simulink model "ejercicio"  (Simulink 5.0)
settings: Solver=ode45  StartTime=0.0  StopTime=75.6  RelTol=1e-3
undefined symbols (not defined in the file): Gama
settings Model: LastModifiedBy=Administrador  RTWOptions="-aEnforceIntegerDowncast=1 -aExtMode=0 -aExtModeTesting=0 -aFoldNonRolledExpr=1 -aForceParamTrailComments=0 -aGenerateComments=1 -aGenerateReport=0 -aIgnoreCustomStorageClasses=1 -aIncDataTypeInIds=0 -aIncHierarchyInIds=0 -aInlineInvariantSignals=0 -aInlinedPrmAccess=\"Literals\" -aLocalBlockOutputs=1 -aLogVarNameModifier=\"rt_\" -aMaxRTWIdLen=31 -aPrefixModelToSubsysFcnNames=1 -aRTWVerbose=1 -aRollThreshold=5 -aShowEliminatedStatements=0"

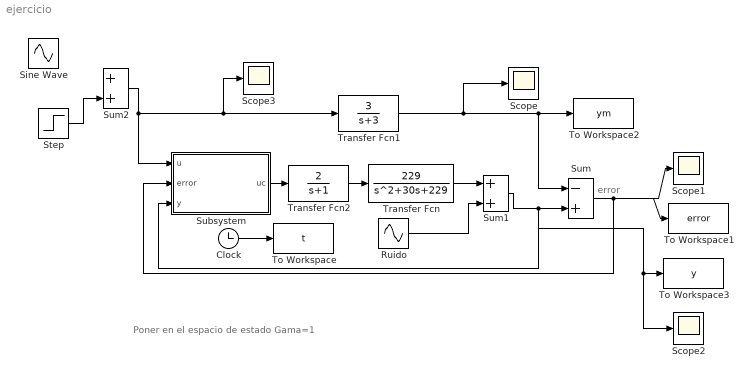
== system ejercicio ==
  note: error
  note: Poner en el espacio de estado
      | Gama=1
  Clock : Clock
      settings: Decimation=10
  "Ruido " : Sin  Amplitude=0.5  Frequency=16.1  SampleTime=0
  Scope{,1..3} (4 alike) : Scope
      Scope2 settings: SaveName=ScopeData2
      Scope3 settings: SaveName=ScopeData5
  Sine Wave : Sin  Amplitude=1.85  Frequency=16  SampleTime=0
  Step : Step  After=2  SampleTime=0
  Subsystem : Subsystem
  Sum : Sum  Inputs=-+  SaturateOnIntegerOverflow=on
  Sum1 : Sum  SaturateOnIntegerOverflow=on
  Sum2 : Sum  SaturateOnIntegerOverflow=on
  To Workspace : ToWorkspace  VariableName=t  SampleTime=-1  SaveFormat=Array
  To Workspace1 : ToWorkspace  VariableName=error  SampleTime=-1  SaveFormat=Array
  To Workspace2 : ToWorkspace  VariableName=ym  SampleTime=-1  SaveFormat=Array
  To Workspace3 : ToWorkspace  VariableName=y  SampleTime=-1  SaveFormat=Array
  Transfer Fcn : TransferFcn  Numerator=[229]  Denominator=[1 30 229]
  Transfer Fcn1 : TransferFcn  Numerator=[3]  Denominator=[1 3]
  Transfer Fcn2 : TransferFcn  Numerator=[2]  Denominator=[1 1]
  wires:
  Clock/1 -> To Workspace/1
  Subsystem/1(uc) -> Transfer Fcn2/1
  Transfer Fcn2/1 -> Transfer Fcn/1
  Step/1 -> Sum2/2
  Sum2/1 -> Subsystem/1(u), Transfer Fcn1/1, Scope3/1
  Transfer Fcn/1 -> Sum1/1
  Sum1/1 -> Sum/2, Subsystem/3("y "), To Workspace3/1, Scope2/1
  Transfer Fcn1/1 -> Sum/1, To Workspace2/1, Scope/1
  Sum/1 -> To Workspace1/1, Subsystem/2("error "), Scope1/1
  "Ruido "/1 -> Sum1/2

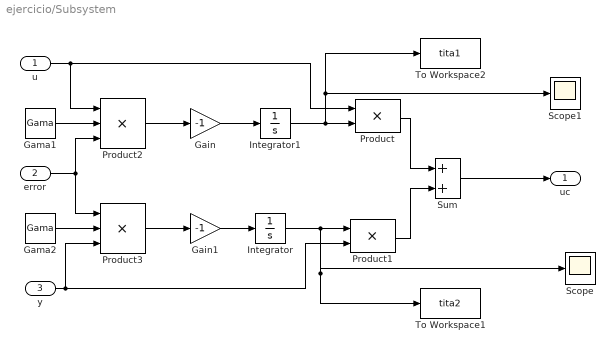
== system ejercicio/Subsystem ==
  u : Inport
  "error " : Inport  Port=2
  "y " : Inport  Port=3
  Gain : Gain  Gain=-1  SaturateOnIntegerOverflow=on
  Gain1 : Gain  Gain=-1  SaturateOnIntegerOverflow=on
  Gama1 : Constant  Value=Gama
  Gama2 : Constant  Value=Gama
  Integrator : Integrator  InitialCondition=-0.65
  Integrator1 : Integrator  InitialCondition=1.14
  Product : Product  SaturateOnIntegerOverflow=on
  Product1 : Product  SaturateOnIntegerOverflow=on
  Product2 : Product  Inputs=3  SaturateOnIntegerOverflow=on
  Product3 : Product  Inputs=3  SaturateOnIntegerOverflow=on
  Scope : Scope
      settings: SaveName=ScopeData3
  Scope1 : Scope
      settings: SaveName=ScopeData4
  Sum : Sum  SaturateOnIntegerOverflow=on
  To Workspace1 : ToWorkspace  VariableName=tita2  SampleTime=-1  SaveFormat=Array
  To Workspace2 : ToWorkspace  VariableName=tita1  SampleTime=-1  SaveFormat=Array
  uc : Outport
  wires:
  "y "/1 -> Product1/2, Product3/3
  Gama2/1 -> Product3/2
  "error "/1 -> Product2/3, Product3/1
  Product3/1 -> Gain1/1
  Gain1/1 -> Integrator/1
  Integrator/1 -> Product1/1, To Workspace1/1, Scope/1
  Product1/1 -> Sum/2
  Product/1 -> Sum/1
  Sum/1 -> uc/1
  Integrator1/1 -> Product/2, To Workspace2/1, Scope1/1
  Gain/1 -> Integrator1/1
  Product2/1 -> Gain/1
  Gama1/1 -> Product2/2
  u/1 -> Product/1, Product2/1
